simulink model "Test_model_Froce"  (R2024a)
settings: Solver=VariableStepAuto  StartTime=0.0  StopTime=inf  RelTol=1e-3
undefined symbols (not defined in the file or in its folder): X, Y, Z
libraries: sm_lib x62, nesl_utility x21, robotcorelib x4, simulink x1
(part 1 of 3)
settings Model: Creator=pimna  LastModifiedBy=TICHABEAR

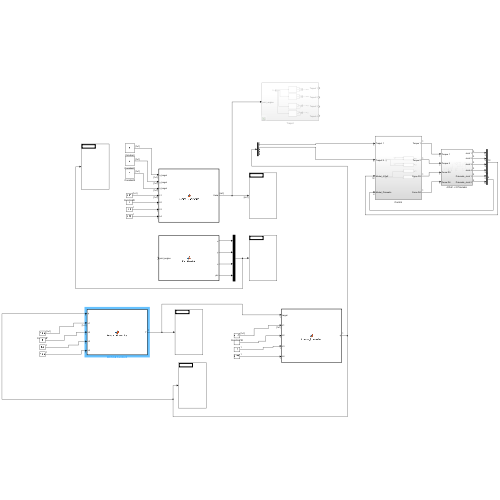
[thumbnail: Simulink's stored preview of the top-level diagram]
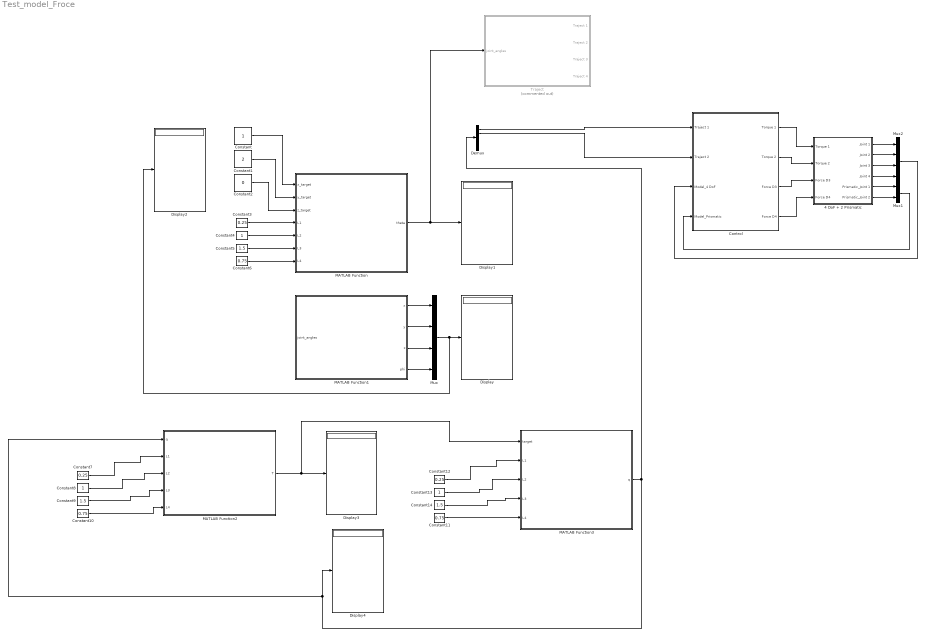
== system Test_model_Froce ==
  4 DoF + 2 Prismatic : Subsystem
  Constant : Constant  VectorParams1D=off  SampleTime=-1
  Constant1 : Constant  Value=2  VectorParams1D=off  SampleTime=-1
  Constant10 : Constant  Value=0.75
  Constant11 : Constant  Value=0.75
  Constant12 : Constant  Value=0.25  VectorParams1D=off  SampleTime=-1
  Constant13 : Constant
  Constant14 : Constant  Value=1.5
  Constant2 : Constant  Value=0  VectorParams1D=off  SampleTime=-1
  Constant3 : Constant  Value=0.25  VectorParams1D=off  SampleTime=-1
  Constant4 : Constant
  Constant5 : Constant  Value=1.5
  Constant6 : Constant  Value=0.75
  Constant7 : Constant  Value=0.25  VectorParams1D=off  SampleTime=-1
  Constant8 : Constant
  Constant9 : Constant  Value=1.5
  Control : Subsystem
  Demux : Demux  Outputs=5
  Display{,1..4} (5 alike) : Display
  MATLAB Function : MATLAB Function  TreatAsAtomicUnit=on
  MATLAB Function1 : MATLAB Function  TreatAsAtomicUnit=on
  MATLAB Function2 : MATLAB Function  TreatAsAtomicUnit=on
  MATLAB Function3 : MATLAB Function  TreatAsAtomicUnit=on
  Mux : Mux
  Mux1 : Mux  Inputs=2
  Mux2 : Mux
  Traject : Subsystem  Commented=on
  wires:
  MATLAB Function1/2(y) -> Mux/2
  MATLAB Function1/4(phi) -> Mux/4
  MATLAB Function1/1(x) -> Mux/1
  MATLAB Function/1(theta) -> Traject/1(joint_angles), Display1/1
  Mux/1 -> Display2/1, Display/1
  MATLAB Function1/3(z) -> Mux/3
  Constant2/1 -> MATLAB Function/3(z_target)
  Constant3/1 -> MATLAB Function/4(L1)
  4 DoF + 2 Prismatic/6(Prismatic_Joint 2) -> Mux1/2
  Constant/1 -> MATLAB Function/1(x_target)
  4 DoF + 2 Prismatic/4(Joint 4) -> Mux2/4
  4 DoF + 2 Prismatic/5(Prismatic_Joint 1) -> Mux1/1
  Mux1/1 -> Control/4(Model_Prismatic)
  4 DoF + 2 Prismatic/1(Joint 1) -> Mux2/1
  Constant1/1 -> MATLAB Function/2(y_target)
  4 DoF + 2 Prismatic/2(Joint 2) -> Mux2/2
  Mux2/1 -> Control/3(Model_4 DoF)
  4 DoF + 2 Prismatic/3(Joint 3) -> Mux2/3
  Control/1(Torque 1) -> 4 DoF + 2 Prismatic/1(Torque 1)
  Control/2(Torque 2) -> 4 DoF + 2 Prismatic/2(Torque 2)
  Demux/1 -> Control/1(Traject 1)
  Demux/2 -> Control/2(Traject 2)
  Control/3(Force D3) -> 4 DoF + 2 Prismatic/3(Force D3)
  Control/4(Force D4) -> 4 DoF + 2 Prismatic/4(Force D4)
  Constant6/1 -> MATLAB Function/7(L4)
  Constant5/1 -> MATLAB Function/6(L3)
  Constant4/1 -> MATLAB Function/5(L2)
  Constant8/1 -> MATLAB Function2/3(L2)
  Constant9/1 -> MATLAB Function2/4(L3)
  Constant10/1 -> MATLAB Function2/5(L4)
  Constant7/1 -> MATLAB Function2/2(L1)
  MATLAB Function2/1(T) -> MATLAB Function3/1(target), Display3/1
  Constant12/1 -> MATLAB Function3/2(L1)
  Constant11/1 -> MATLAB Function3/5(L4)
  Constant14/1 -> MATLAB Function3/4(L3)
  Constant13/1 -> MATLAB Function3/3(L2)
  MATLAB Function3/1(q) -> MATLAB Function2/1(q), Display4/1, Demux/1
